simulink model "first"  (R2023b)
settings: Solver=FixedStepAuto  StartTime=0.0  StopTime=15  FixedStep=0.0001  RelTol=1e-3
undefined symbols (not defined in the file or in its folder): A, B_1, B_2, C, D, K_1, x_0
settings Model: Creator=evdokiiagalkina  LastModifiedBy=evdokiiagalkina

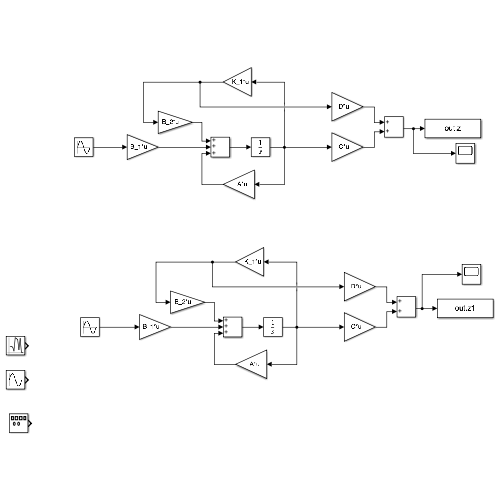
[thumbnail: Simulink's stored preview of the top-level diagram]
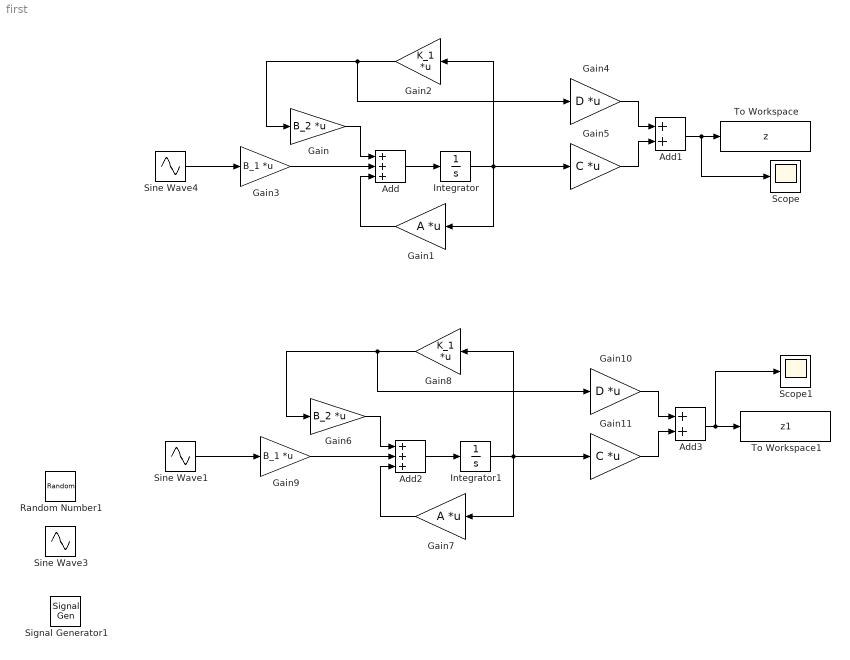
== system first ==
  Add : Sum  Inputs=+++
  Add1 : Sum
  Add2 : Sum  Inputs=+++
  Add3 : Sum
  Gain : Gain  Gain=B_2  Multiplication=Matrix(K*u)
  Gain1 : Gain  Gain=A  Multiplication=Matrix(K*u)
  Gain10 : Gain  Gain=D  Multiplication=Matrix(K*u)
  Gain11 : Gain  Gain=C  Multiplication=Matrix(K*u)
  Gain2 : Gain  Gain=K_1  Multiplication=Matrix(K*u)
  Gain3 : Gain  Gain=B_1  Multiplication=Matrix(K*u)
  Gain4 : Gain  Gain=D  Multiplication=Matrix(K*u)
  Gain5 : Gain  Gain=C  Multiplication=Matrix(K*u)
  Gain6 : Gain  Gain=B_2  Multiplication=Matrix(K*u)
  Gain7 : Gain  Gain=A  Multiplication=Matrix(K*u)
  Gain8 : Gain  Gain=K_1  Multiplication=Matrix(K*u)
  Gain9 : Gain  Gain=B_1  Multiplication=Matrix(K*u)
  Integrator : Integrator  InitialCondition=x_0
  Integrator1 : Integrator  InitialCondition=x_0
  Random Number1 : RandomNumber  Mean=1  SampleTime=0.001
  Scope : Scope
  Scope1 : Scope
  Signal Generator1 : SignalGenerator  WaveForm=square  Amplitude=100  Units=rad/sec
  Sine Wave1 : Sin  Amplitude=100  Frequency=20  SampleTime=0
  Sine Wave3 : Sin  Amplitude=100  SampleTime=0
  Sine Wave4 : Sin  Amplitude=100  SampleTime=0
  To Workspace : ToWorkspace  VariableName=z  SaveFormat=Timeseries  SampleTime=-1
  To Workspace1 : ToWorkspace  VariableName=z1  SaveFormat=Timeseries  SampleTime=-1
  wires:
  Add3/1 -> Scope1/1, To Workspace1/1
  Gain8/1 -> Gain10/1, Gain6/1
  Gain6/1 -> Add2/1
  Gain1/1 -> Add/3
  Gain7/1 -> Add2/3
  Gain9/1 -> Add2/2
  Add1/1 -> Scope/1, To Workspace/1
  Gain11/1 -> Add3/2
  Add2/1 -> Integrator1/1
  Gain5/1 -> Add1/2
  Gain2/1 -> Gain4/1, Gain/1
  Integrator/1 -> Gain1/1, Gain5/1, Gain2/1
  Integrator1/1 -> Gain7/1, Gain11/1, Gain8/1
  Gain10/1 -> Add3/1
  Add/1 -> Integrator/1
  Gain4/1 -> Add1/1
  Gain3/1 -> Add/2
  Gain/1 -> Add/1
  Sine Wave4/1 -> Gain3/1
  Sine Wave1/1 -> Gain9/1
